simulink model "q3"  (R2024a)
settings: Solver=FixedStepAuto  StartTime=0.0  StopTime=10.0  FixedStep=0.1  RelTol=1e-3
settings Model: ExtModeTrigDuration=2  Creator=amir  LastModifiedBy=amir
settings SolverCC: AutoInsertRateTranBlk=on
settings OptimizationCC: DefaultParameterBehavior=Inlined  UseDivisionForNetSlopeComputation=on  GainParamInheritBuiltInType=on  UseFloatMulNetSlope=on  InlineInvariantSignals=on  PassReuseOutputArgsAs=Individual arguments  ZeroExternalMemoryAtStartup=off  ZeroInternalMemoryAtStartup=off  NoFixptDivByZeroProtection=on  EfficientFloat2IntCast=on  LifeSpan=1  MaxStackSize=64  OptimizeBlockOrder=speed  DifferentSizesBufferReuse=on  EfficientTunableParamExpr=on
settings DebuggingCC: ParameterTunabilityLossMsg=error
settings HardwareCC: ProdBitPerInt=16  ProdBitPerPointer=16  ProdBitPerSizeT=16  ProdBitPerPtrDiffT=16  ProdLargestAtomicFloat=None  ProdWordSize=8  ProdLongLongMode=on  ProdHWDeviceType=Atmel->AVR
settings SFSimCC: MATLABDynamicMemAlloc=off
settings RTWCC: Description=Embedded Coder  SystemTargetFile=ert.tlc  HardwareBoard=Arduino Uno  TemplateMakefile=ert_default_tmf  Toolchain=Arduino AVR  BuildConfiguration=Faster Runs
settings CodeAppCC: ForceParamTrailComments=on  IgnoreCustomStorageClasses=off  OperatorAnnotations=on  SimulinkDataObjDesc=on  SFDataObjDesc=on  CustomSymbolStrGlobalVar=rt$N$M  CustomSymbolStrType=$N$M  CustomSymbolStrFcn=$N$M$F  CustomSymbolStrMacro=$N$M  InsertBlockDesc=on
settings ERTTargetCC: IncludeMdlTerminateFcn=off  CombineSignalStateStructs=on  SupportComplex=off  SupportNonInlinedSFcns=on  ExtModeTransport=3  ExtModeStaticAlloc=on  ExtModeAutomaticAllocSize=off  ExtModeStaticAllocSize=250  ExtModeMexFile=ext_xcp  ExtModeIntrfLevel=Level2 - Open  InlinedParameterPlacement=NonHierarchical  ERTFilePackagingFormat=CompactWithDataFile
settings ConfigComp: CovEnable=on  RecordCoverage=on  CovModelRefEnable=on

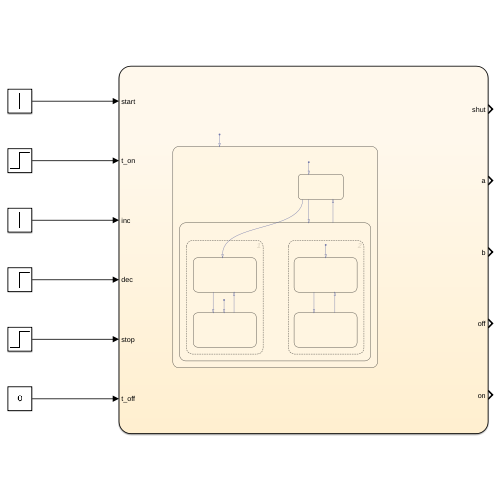
[thumbnail: Simulink's stored preview of the top-level diagram]
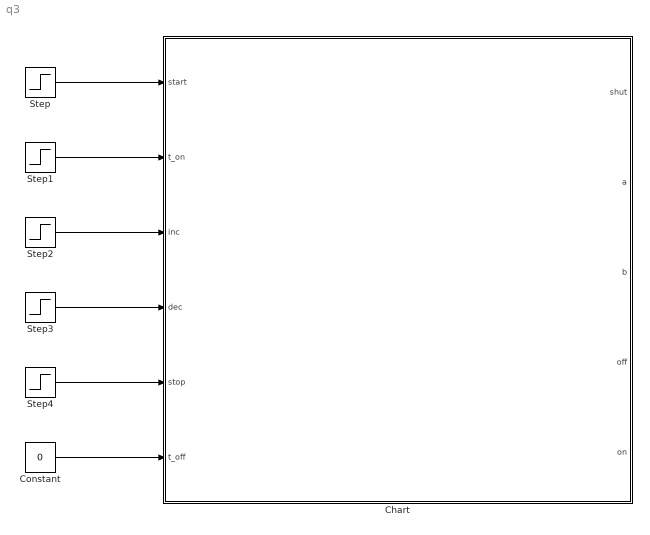
== system q3 ==
  Chart : Stateflow chart  TreatAsAtomicUnit=on
  Constant : Constant  Value=0
  Step : Step  SampleTime=0
  Step1 : Step  Time=1.1  SampleTime=0
  Step2 : Step  Time=1.2  SampleTime=0
  Step3 : Step  Time=1.3  SampleTime=0
  Step4 : Step  Time=1.4  SampleTime=0
  wires:
  Step/1 -> Chart/1(start)
  Step1/1 -> Chart/2(t_on)
  Step2/1 -> Chart/3(inc)
  Step3/1 -> Chart/4(dec)
  Step4/1 -> Chart/5(stop)
  Constant/1 -> Chart/6(t_off)

== stateflow chart q3/Chart ==
  state Alarm
    state Shut
    state Op
      state Mode [parallel]
        settings: executionOrder=1
        state On
        state Off
        On -> Off : [t_off]{off=1; on=0;}
        Off -> On : [t_on]{on=1; off=0;}
        (default) -> Off : {off=1;}
      state Vol [parallel]
        settings: executionOrder=2
        state a
        state b
        (default) -> a : {a=1;}
        a -> b : [inc]{a=0; b=1;}
        b -> a : [dec]{a=1; b=0;}
    (default) -> Shut : {shut=1; a=0; b=0; on=0; off=0;}
    Shut -> On [order 2] : [t_on]{shut=0; on=1;}
    Shut -> Op [order 1] : [start]{shut=0;}
    Op -> Shut : [stop]{shut=1; a=0; b=0; on=0; off=0;}
  (default) -> Alarm
  data: start input; t_on input; inc input; dec input; stop input; t_off input; shut output; a output; b output; off output; on output
